simulink model "PD_Control"  (R2021b)
settings: Solver=VariableStepAuto  StartTime=0.0  StopTime=10  RelTol=1e-3
undefined symbols (not defined in the file): q_d, q_dq_init
settings Model: Creator=Yafei Ou  LastModifiedBy=Kirill

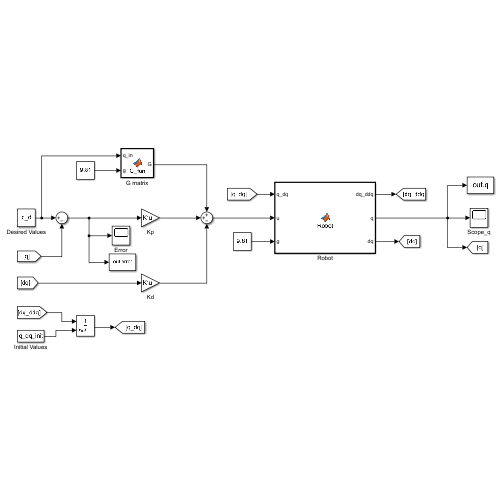
[thumbnail: Simulink's stored preview of the top-level diagram]
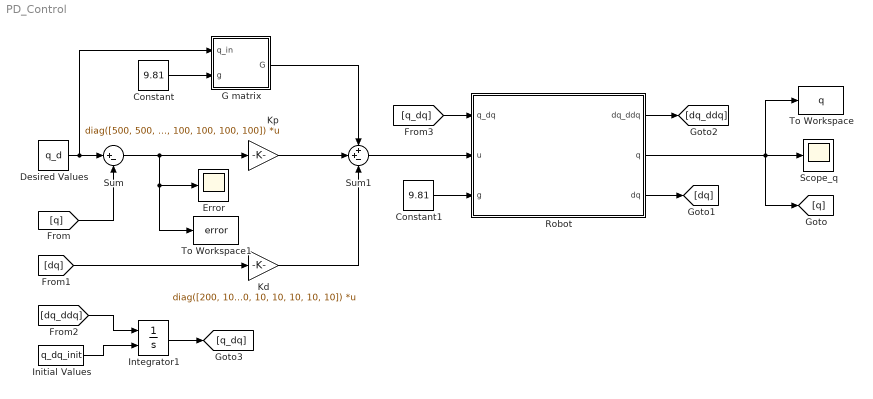
== system PD_Control ==
  Constant : Constant  Value=9.81
  Constant1 : Constant  Value=9.81
  Desired Values : Constant  Value=q_d
  Error : Scope
  G matrix : MATLAB Function  TreatAsAtomicUnit=on
  Initial Values : Constant  Value=q_dq_init
  Integrator1 : Integrator  InitialConditionSource=external
  Kd : Gain  Gain=diag([200, 100, 10, 10, 10, 10, 10])  Multiplication=Matrix(K*u)
  Kp : Gain  Gain=diag([500, 500, 100, 100, 100, 100, 100])  Multiplication=Matrix(K*u)
  Robot : MATLAB Function  TreatAsAtomicUnit=on
  Scope_q : Scope
  Sum : Sum  Inputs=|+-
  Sum1 : Sum  Inputs=++-
  To Workspace : ToWorkspace  VariableName=q  SampleTime=-1
      settings: Save2DSignal=2-D array (concatenate along first dimension)
  To Workspace1 : ToWorkspace  VariableName=error  SampleTime=-1
      settings: Save2DSignal=2-D array (concatenate along first dimension)
  wires:
  Desired Values/1 -> G matrix/1(q_in), Sum/1
  Kd/1 -> Sum1/3
  Kp/1 -> Sum1/2
  G matrix/1(G) -> Sum1/1
  Sum1/1 -> Robot/2(u)
  Constant/1 -> G matrix/2(g)
  Sum/1 -> Kp/1, To Workspace1/1, Error/1
  Constant1/1 -> Robot/3(g)
  [q] -> Sum/2
  [dq] -> Kd/1
  Robot/3(dq) -> [dq]
  Robot/2(q) -> To Workspace/1, Scope_q/1, [q]
  Robot/1(dq_ddq) -> [dq_ddq]
  [dq_ddq] -> Integrator1/1
  Initial Values/1 -> Integrator1/2
  Integrator1/1 -> [q_dq]
  [q_dq] -> Robot/1(q_dq)

== matlab function PD_Control/G matrix ==
  data: q_in input; G output; g input
function G = G_fun(q_in,g)
%G_fun
%    G = G_fun(Q1,Q2,Q3,Q4,Q5,Q6,Q7,g)

%    This function was generated by the Symbolic Math Toolbox version 9.0.
%    14-Apr-2022 19:25:58

q1 = q_in(1); 
q2 = q_in(2); 
q3 = q_in(3);
q4 = q_in(4);
q5 = q_in(5);
q6 = q_in(6); 
q7 = q_in(7);

t2 = cos(q2);
t3 = cos(q3);
t4 = cos(q4);
t5 = cos(q5);
t6 = cos(q6);
t7 = cos(q7);
t8 = sin(q2);
t9 = sin(q3);
t10 = sin(q4);
t11 = sin(q5);
t12 = sin(q6);
t13 = sin(q7);
et1 = g.*t2.*3.45360925e-2-g.*t8.*4.3163130985+g.*t2.*t3.*5.5242e-3-g.*t2.*t9.*1.85444563e-1;
et2 = g.*t4.*t8.*(-2.002662146)-g.*t8.*t10.*5.2231e-4-g.*t2.*t3.*t4.*5.2231e-4+g.*t2.*t3.*t10.*2.002662146;
et3 = g.*t2.*t5.*t9.*(-1.01250325e-1)-g.*t4.*t6.*t8.*1.532971099999998e-3+g.*t2.*t9.*t11.*1.705e-4-g.*t5.*t8.*t10.*1.705e-4;
et4 = g.*t4.*t8.*t12.*1.6600955e-3-g.*t8.*t10.*t11.*1.01250325e-1-g.*t2.*t3.*t4.*t5.*1.705e-4-g.*t2.*t3.*t4.*t11.*1.01250325e-1;
et5 = g.*t2.*t3.*t6.*t10.*1.532971099999998e-3-g.*t2.*t5.*t7.*t9.*8.2343968e-3-g.*t2.*t3.*t10.*t12.*1.6600955e-3+g.*t2.*t6.*t9.*t11.*1.6600955e-3;
et6 = g.*t2.*t5.*t9.*t13.*(-1.22807312e-2)-g.*t5.*t6.*t8.*t10.*1.6600955e-3-g.*t4.*t7.*t8.*t12.*1.22807312e-2+g.*t2.*t9.*t11.*t12.*1.532971099999998e-3;
et7 = g.*t5.*t8.*t10.*t12.*(-1.532971099999998e-3)-g.*t7.*t8.*t10.*t11.*8.2343968e-3+g.*t4.*t8.*t12.*t13.*8.2343968e-3-g.*t8.*t10.*t11.*t13.*1.22807312e-2;
et8 = g.*t2.*t3.*t4.*t5.*t6.*(-1.6600955e-3)-g.*t2.*t3.*t4.*t5.*t12.*1.532971099999998e-3-g.*t2.*t3.*t4.*t7.*t11.*8.2343968e-3-g.*t2.*t3.*t4.*t11.*t13.*1.22807312e-2;
et9 = g.*t2.*t3.*t7.*t10.*t12.*1.22807312e-2-g.*t2.*t6.*t7.*t9.*t11.*1.22807312e-2+g.*t5.*t6.*t7.*t8.*t10.*1.22807312e-2-g.*t2.*t3.*t10.*t12.*t13.*8.2343968e-3;
et10 = g.*t2.*t6.*t9.*t11.*t13.*8.2343968e-3-g.*t5.*t6.*t8.*t10.*t13.*8.2343968e-3+g.*t2.*t3.*t4.*t5.*t6.*t7.*1.22807312e-2-g.*t2.*t3.*t4.*t5.*t6.*t13.*8.2343968e-3;
et11 = g.*t3.*t8.*(-1.85444563e-1)-g.*t8.*t9.*5.5242e-3-g.*t3.*t5.*t8.*1.01250325e-1+g.*t4.*t8.*t9.*5.2231e-4;
et12 = g.*t3.*t8.*t11.*1.705e-4-g.*t8.*t9.*t10.*2.002662146-g.*t3.*t5.*t7.*t8.*8.2343968e-3+g.*t4.*t5.*t8.*t9.*1.705e-4;
et13 = g.*t3.*t6.*t8.*t11.*1.6600955e-3-g.*t3.*t5.*t8.*t13.*1.22807312e-2+g.*t4.*t8.*t9.*t11.*1.01250325e-1-g.*t6.*t8.*t9.*t10.*1.532971099999998e-3;
et14 = g.*t3.*t8.*t11.*t12.*1.532971099999998e-3+g.*t8.*t9.*t10.*t12.*1.6600955e-3+g.*t4.*t5.*t6.*t8.*t9.*1.6600955e-3-g.*t3.*t6.*t7.*t8.*t11.*1.22807312e-2;
et15 = g.*t4.*t5.*t8.*t9.*t12.*1.532971099999998e-3+g.*t4.*t7.*t8.*t9.*t11.*8.2343968e-3+g.*t3.*t6.*t8.*t11.*t13.*8.2343968e-3+g.*t4.*t8.*t9.*t11.*t13.*1.22807312e-2;
et16 = g.*t7.*t8.*t9.*t10.*t12.*(-1.22807312e-2)+g.*t8.*t9.*t10.*t12.*t13.*8.2343968e-3-g.*t4.*t5.*t6.*t7.*t8.*t9.*1.22807312e-2+g.*t4.*t5.*t6.*t8.*t9.*t13.*8.2343968e-3;
et17 = g.*t2.*t4.*5.2231e-4-g.*t2.*t10.*2.002662146+g.*t2.*t4.*t5.*1.705e-4+g.*t3.*t4.*t8.*2.002662146;
et18 = g.*t2.*t4.*t11.*1.01250325e-1-g.*t2.*t6.*t10.*1.532971099999998e-3+g.*t3.*t8.*t10.*5.2231e-4+g.*t2.*t10.*t12.*1.6600955e-3;
et19 = g.*t2.*t4.*t5.*t6.*1.6600955e-3+g.*t3.*t4.*t6.*t8.*1.532971099999998e-3+g.*t2.*t4.*t5.*t12.*1.532971099999998e-3+g.*t2.*t4.*t7.*t11.*8.2343968e-3;
et20 = g.*t3.*t5.*t8.*t10.*1.705e-4-g.*t3.*t4.*t8.*t12.*1.6600955e-3+g.*t2.*t4.*t11.*t13.*1.22807312e-2-g.*t2.*t7.*t10.*t12.*1.22807312e-2;
et21 = g.*t3.*t8.*t10.*t11.*1.01250325e-1+g.*t2.*t10.*t12.*t13.*8.2343968e-3-g.*t2.*t4.*t5.*t6.*t7.*1.22807312e-2+g.*t2.*t4.*t5.*t6.*t13.*8.2343968e-3;
et22 = g.*t3.*t5.*t6.*t8.*t10.*1.6600955e-3+g.*t3.*t4.*t7.*t8.*t12.*1.22807312e-2+g.*t3.*t5.*t8.*t10.*t12.*1.532971099999998e-3+g.*t3.*t7.*t8.*t10.*t11.*8.2343968e-3;
et23 = g.*t3.*t4.*t8.*t12.*t13.*(-8.2343968e-3)+g.*t3.*t8.*t10.*t11.*t13.*1.22807312e-2-g.*t3.*t5.*t6.*t7.*t8.*t10.*1.22807312e-2+g.*t3.*t5.*t6.*t8.*t10.*t13.*8.2343968e-3;
et24 = g.*t2.*t5.*t10.*1.01250325e-1+g.*t5.*t8.*t9.*1.705e-4-g.*t2.*t10.*t11.*1.705e-4+g.*t8.*t9.*t11.*1.01250325e-1;
et25 = g.*t3.*t4.*t5.*t8.*(-1.01250325e-1)+g.*t2.*t5.*t7.*t10.*8.2343968e-3+g.*t3.*t4.*t8.*t11.*1.705e-4+g.*t5.*t6.*t8.*t9.*1.6600955e-3;
et26 = g.*t2.*t6.*t10.*t11.*(-1.6600955e-3)+g.*t2.*t5.*t10.*t13.*1.22807312e-2+g.*t5.*t8.*t9.*t12.*1.532971099999998e-3-g.*t2.*t10.*t11.*t12.*1.532971099999998e-3;
et27 = g.*t7.*t8.*t9.*t11.*8.2343968e-3+g.*t8.*t9.*t11.*t13.*1.22807312e-2-g.*t3.*t4.*t5.*t7.*t8.*8.2343968e-3+g.*t3.*t4.*t6.*t8.*t11.*1.6600955e-3;
et28 = g.*t3.*t4.*t5.*t8.*t13.*(-1.22807312e-2)-g.*t5.*t6.*t7.*t8.*t9.*1.22807312e-2+g.*t2.*t6.*t7.*t10.*t11.*1.22807312e-2+g.*t3.*t4.*t8.*t11.*t12.*1.532971099999998e-3;
et29 = g.*t5.*t6.*t8.*t9.*t13.*8.2343968e-3-g.*t2.*t6.*t10.*t11.*t13.*8.2343968e-3-g.*t3.*t4.*t6.*t7.*t8.*t11.*1.22807312e-2+g.*t3.*t4.*t6.*t8.*t11.*t13.*8.2343968e-3;
et30 = g.*t2.*t4.*t6.*(-1.6600955e-3)-g.*t2.*t4.*t12.*1.532971099999998e-3+g.*t2.*t4.*t6.*t7.*1.22807312e-2+g.*t2.*t5.*t6.*t10.*1.532971099999998e-3;
et31 = g.*t2.*t4.*t6.*t13.*(-8.2343968e-3)-g.*t3.*t6.*t8.*t10.*1.6600955e-3-g.*t2.*t5.*t10.*t12.*1.6600955e-3-g.*t3.*t8.*t10.*t12.*1.532971099999998e-3;
et32 = g.*t6.*t8.*t9.*t11.*1.532971099999998e-3-g.*t8.*t9.*t11.*t12.*1.6600955e-3-g.*t3.*t4.*t5.*t6.*t8.*1.532971099999998e-3+g.*t3.*t4.*t5.*t8.*t12.*1.6600955e-3;
et33 = g.*t3.*t6.*t7.*t8.*t10.*1.22807312e-2+g.*t2.*t5.*t7.*t10.*t12.*1.22807312e-2-g.*t3.*t6.*t8.*t10.*t13.*8.2343968e-3-g.*t2.*t5.*t10.*t12.*t13.*8.2343968e-3;
et34 = g.*t7.*t8.*t9.*t11.*t12.*1.22807312e-2-g.*t8.*t9.*t11.*t12.*t13.*8.2343968e-3-g.*t3.*t4.*t5.*t7.*t8.*t12.*1.22807312e-2+g.*t3.*t4.*t5.*t8.*t12.*t13.*8.2343968e-3;
et35 = g.*t2.*t4.*t7.*t12.*(-8.2343968e-3)-g.*t5.*t7.*t8.*t9.*1.22807312e-2+g.*t2.*t7.*t10.*t11.*1.22807312e-2-g.*t2.*t4.*t12.*t13.*1.22807312e-2;
et36 = g.*t5.*t8.*t9.*t13.*8.2343968e-3-g.*t2.*t10.*t11.*t13.*8.2343968e-3+g.*t2.*t5.*t6.*t7.*t10.*8.2343968e-3-g.*t3.*t4.*t7.*t8.*t11.*1.22807312e-2;
et37 = g.*t2.*t5.*t6.*t10.*t13.*1.22807312e-2+g.*t3.*t4.*t8.*t11.*t13.*8.2343968e-3-g.*t3.*t7.*t8.*t10.*t12.*8.2343968e-3+g.*t6.*t7.*t8.*t9.*t11.*8.2343968e-3;
et38 = g.*t3.*t8.*t10.*t12.*t13.*(-1.22807312e-2)+g.*t6.*t8.*t9.*t11.*t13.*1.22807312e-2-g.*t3.*t4.*t5.*t6.*t7.*t8.*8.2343968e-3-g.*t3.*t4.*t5.*t6.*t8.*t13.*1.22807312e-2;
G = [0.0;et1+et2+et3+et4+et5+et6+et7+et8+et9+et10;et11+et12+et13+et14+et15+et16;et17+et18+et19+et20+et21+et22+et23;et24+et25+et26+et27+et28+et29;et30+et31+et32+et33+et34;et35+et36+et37+et38];

== matlab function PD_Control/Robot ==
  data: q_dq input; dq_ddq output; u input; q output; dq output; g input
function [dq_ddq,q,dq] = Robot(q_dq,u,g)
    q = q_dq(1:length(q_dq)/2);
    dq = q_dq(length(q_dq)/2+1:length(q_dq));
    g_num = g;

    M = M_fun(q);
    C = C_fun(q,dq);
    G = G_fun(q,g_num);

    ddq = M\(u - C - G);
    
    dq_ddq = [dq;ddq];

end
